simulink model "lab2_sim_2"  (R2018b)
settings: Solver=VariableStepAuto  StartTime=0.0  StopTime=10.0  RelTol=1e-3
values from neighbouring files (symbols this model uses):
  snr = SNR_dB(i)    [sim_code.m]    (also in sim_code2.m)
libraries: commrandsrc3 x1
settings Model: Creator=DSP_08  LastModifiedBy=DSP_08

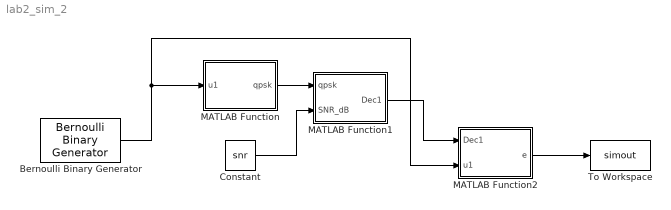
== system lab2_sim_2 ==
  Bernoulli Binary Generator : commrandsrc3/Bernoulli Binary Generator  ProbabilityOfZero=0.5  SeedSource=Auto  Seed=0  SampleTime=1  SamplesPerFrame=10000  OutputDataType=double  SimulateUsing=Interpreted execution
  Constant : Constant  Value=snr
  MATLAB Function : MATLAB Function  TreatAsAtomicUnit=on
  MATLAB Function1 : MATLAB Function  TreatAsAtomicUnit=on
  MATLAB Function2 : MATLAB Function  TreatAsAtomicUnit=on
  To Workspace : ToWorkspace  VariableName=simout  SampleTime=-1
      settings: Save2DSignal=2-D array (concatenate along first dimension)
  wires:
  MATLAB Function/1(qpsk) -> MATLAB Function1/1(qpsk)
  Constant/1 -> MATLAB Function1/2(SNR_dB)
  MATLAB Function1/1(Dec1) -> MATLAB Function2/1(Dec1)
  Bernoulli Binary Generator/1 -> MATLAB Function2/2(u1), MATLAB Function/1(u1)
  MATLAB Function2/1(e) -> To Workspace/1

== matlab function lab2_sim_2/MATLAB Function1 ==
  data: qpsk input; Dec1 output; SNR_dB input
function Dec1 = fcn(qpsk,SNR_dB)

    N = length(qpsk);
    h = complex(randn(1,N),randn(1,N));
    noise = complex(randn(1,N),randn(1,N));
    y = zeros(1,N) + 1j*zeros(1,N);
    Dec1 = zeros(1,N) + 1j*zeros(1,N);
    SNR_lin = 10^(SNR_dB/10);
    sigma = 1/sqrt(SNR_lin);
    
    y = h.*qpsk + sigma*noise;
    Dec1 = y./h;
    
end

== matlab function lab2_sim_2/MATLAB Function ==
  data: u1 input; qpsk output
function qpsk = fcn(u1)

    X = transpose(u1);
    N = length(X);
    qpsk = zeros(1,N/2) + 1j*zeros(1,N/2);;
    n = 1;
    for i = 1:2:N
        if (X(i) == 0) && (X(i+1) == 0)
            qpsk(n) = (1+1j)/sqrt(2);
        elseif (X(i) == 0) && (X(i+1) == 1)
            qpsk(n) = (-1+1j)/sqrt(2);
        elseif (X(i) == 1) && (X(i+1) == 0)
            qpsk(n) = (-1-1j)/sqrt(2);
        elseif (X(i) == 1) && (X(i+1) == 1)
            qpsk(n) = (1-1j)/sqrt(2);
        end
    n = n+1;
    end
end

== matlab function lab2_sim_2/MATLAB Function2 ==
  data: Dec1 input; e output; u1 input
function e = fcn(Dec1,u1)

    N = length(Dec1);
    X = transpose(u1);
    X_rcvd = zeros(1,N*2);
    
    n = 1;
    for j = 1:N
        if (real(Dec1(j))>0) && (imag(Dec1(j))>0)
            X_rcvd(n) = 0;
            X_rcvd(n+1) = 0;
        elseif (real(Dec1(j))<0) && (imag(Dec1(j))>0)
            X_rcvd(n) = 0;
            X_rcvd(n+1) = 1;
        elseif (real(Dec1(j))<0) && (imag(Dec1(j))<0)
            X_rcvd(n) = 1;
            X_rcvd(n+1) = 0;
        elseif (real(Dec1(j))>0) && (imag(Dec1(j))<0)
            X_rcvd(n) = 1;
            X_rcvd(n+1) = 1;
        end
        n = n+2;
    end
    e = sum(abs(X-X_rcvd))/(2*N);
end
